simulink model "Control_AC_InducationMotor_P2"  (R2021a)
settings: Solver=VariableStepAuto  StartTime=0.0  StopTime=0.8  MaxStep=1e-6  RelTol=1e-3
libraries: spsIdealSwitchLib x4, spsDCVoltageSourceLib x2, spsCurrentMeasurementLib x1, spsSeriesRLCBranchLib x1, spsTriangleGeneratorLib x1, spsVoltageMeasurementLib x1, spspowerguiLib x1
settings Model: Creator=Shashwat M.A  LastModifiedBy=Shashwat M.A
settings DataIOCC: ReturnWorkspaceOutputs=off

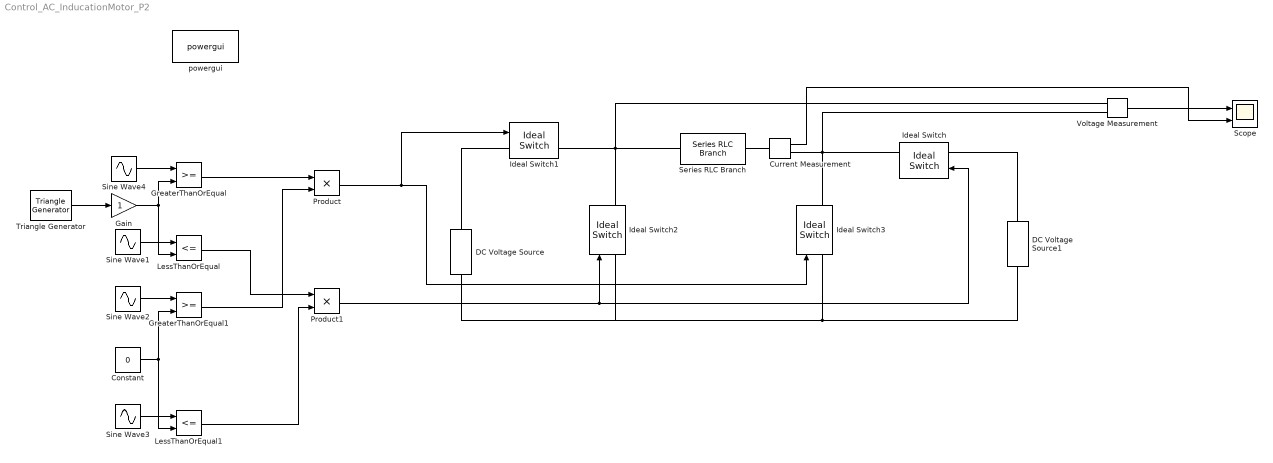
== system Control_AC_InducationMotor_P2 ==
  Constant : Constant  Value=0
  Current Measurement : spsCurrentMeasurementLib/Current Measurement  PhasorSimulation=off  OutputType=Complex  PSBequivalent=0
  DC Voltage Source : spsDCVoltageSourceLib/DC Voltage Source  Amplitude=100  Measurements=None
  DC Voltage Source1 : spsDCVoltageSourceLib/DC Voltage Source  Amplitude=100  Measurements=None
  Gain : Gain
  GreaterThanOrEqual : RelationalOperator  OutDataTypeStr=boolean  RndMeth=Simplest
  GreaterThanOrEqual1 : RelationalOperator  OutDataTypeStr=boolean  RndMeth=Simplest
  Ideal Switch{,1..3} (4 alike) : spsIdealSwitchLib/Ideal Switch  Ron=0.001  Lon=0  IC=0  Rs=1e5  Cs=inf  Measurements=on
  LessThanOrEqual : RelationalOperator  Operator=<=  OutDataTypeStr=boolean  RndMeth=Simplest
  LessThanOrEqual1 : RelationalOperator  Operator=<=  OutDataTypeStr=boolean  RndMeth=Simplest
  Product : Product
  Product1 : Product
  Scope : Scope  NumInputPorts=2
  Series RLC Branch : spsSeriesRLCBranchLib/Series RLC Branch  LConnTagsString=__new0  RConnTagsString=__new0  BranchType=R  Resistance=10  Inductance=1e-3  SetiL0=off  InitialCurrent=0  Capacitance=1e-6  Setx0=off  InitialVoltage=0  Measurements=None
  Sine Wave{1..4} (4 alike) : Sin  Frequency=50  SampleTime=0
  Triangle Generator : spsTriangleGeneratorLib/Triangle Generator  Freq=1050  Phase=180  Ts=0
  Voltage Measurement : spsVoltageMeasurementLib/Voltage Measurement  PhasorSimulation=off  OutputType=Complex  PSBequivalent=0
  powergui : spspowerguiLib/powergui  Priority=1  SimulationMode=Continuous  SampleTime=50e-6  frequency=60  Iterations=50  frequencyindice=0  Pbase=100e6  ErrMax=1e-4  UnitsV=kV  UnitsW=MW  buscounter=0  FunctionMessages=off  echomessages=off  EnableUseOfTLC=off  CurrentSourceSwitches=off  DisableSnubberDevices=off  DisableRonSwitches=off  DisableVfSwitches=off  DisplayEquations=off  AutomaticDiscreteSolvers=off  SolverType=Tustin/Backward Euler (TBE)  Interpol=off  ExternalGateDelay=off  methode=off  Ts=100  x0status=blocks  SPID=on  SwTol=0  HookPort=off  NonlinearTolerance=1e-4  nMaxIteration=100  ContinueOnMaxIteration=off  RestoreLinks=warning  ResistiveCurrentMeasurement=off  Frange=[0:2:500]  Ylog=off  Xlog=on  ShowGrid=off  save=off  variable=ZData  structure=0  ZoomFFT=off  StartTime=0.0  cycles=1  DisplayStyle=1  fundamental=60  FreqAxis=off  MaxFrequency=1000  frequencyindicesteady=1  RmsSteady=1  display=off
  wires:
  Voltage Measurement/1 -> Scope/1
  Current Measurement/1 -> Scope/2
  GreaterThanOrEqual/1 -> Product/1
  GreaterThanOrEqual1/1 -> Product/2
  Product/1 -> Ideal Switch3/1, Ideal Switch1/1
  Product1/1 -> Ideal Switch/1, Ideal Switch2/1
  LessThanOrEqual/1 -> Product1/1
  LessThanOrEqual1/1 -> Product1/2
  Sine Wave4/1 -> GreaterThanOrEqual/1
  Sine Wave1/1 -> LessThanOrEqual/1
  Constant/1 -> GreaterThanOrEqual1/2, LessThanOrEqual1/2
  Sine Wave3/1 -> LessThanOrEqual1/1
  Triangle Generator/1 -> Gain/1
  Gain/1 -> GreaterThanOrEqual/2, LessThanOrEqual/2
  Sine Wave2/1 -> GreaterThanOrEqual1/1
  connections:
  DC Voltage Source/RConn1 -- Ideal Switch1/LConn1
  Series RLC Branch/LConn1 -- Ideal Switch2/RConn1 -- Voltage Measurement/LConn1 -- Ideal Switch1/RConn1
  Ideal Switch/RConn1 -- Voltage Measurement/LConn2 -- Current Measurement/RConn1 -- Ideal Switch3/RConn1
  Ideal Switch/LConn1 -- DC Voltage Source1/RConn1
  DC Voltage Source1/LConn1 -- Ideal Switch2/LConn1 -- DC Voltage Source/LConn1 -- Ideal Switch3/LConn1
  Current Measurement/LConn1 -- Series RLC Branch/RConn1
